simulink model "Simulator1"  (R2024a)
settings: Solver=VariableStepAuto  StartTime=0.0  StopTime=inf  RelTol=1e-5
values from neighbouring files (symbols this model uses):
  I = [3000 0 0 ... (first row only)    [Constants_gui.m]    (also in constants.m; mbi.m = [15, .25, .20; set_up_HW7.m = I-Id; setupConstantRateSDA.m)
  invI = inv(I)    [Constants_gui.m]    (also in constants.m; mbi.m; set_up_HW7.m; setupConstantRateSDA.m)
  q_init = q_init/norm(q_init)    [Constants_gui.m]    (also in constants.m = [-0.5 -0.5 -0.5 0.5]; mbi.m = [0 0 0 1]'; set_up_HW7.m = [0 0 0 1]'; setupConstantRateSDA.m)
  wbn_init = pi/30*[0 0 0]'    [Constants_gui.m]    (also in constants.m = pi/180 * [0.1; 0.2; 0.15]; mbi.m = [0 0 0]'; set_up_HW7.m = pi/30*[0 0 .01]'; setupConstantRateSDA.m)
  wn = 0.01    [Constants_gui.m]    (also in constants.m = 0.05; setupConstantRateSDA.m = 0.05)
  zet = .7071    (= 0.7071)    [Constants_gui.m]    (also in constants.m; setupConstantRateSDA.m)
undefined symbols (not defined in the file or in its folder): w_init
libraries: sharedtransform x5, aerolibutil x5, sharedutil x3, simulink x2, dspinverses x1
(part 4 of 4)

== system Simulator1/Mode 4: Slew1/ACS/Free Rigid Body /Quaternion Integration ==
  w_Body : Inport
  Integrator1 : Integrator  InitialCondition=q_init
  q_normalize : Subsystem
  qderiv : Subsystem
  q_I_Body : Outport
  wires:
  w_Body/1 -> qderiv/1(w)
  q_normalize/1(q_out) -> qderiv/2(q), q_I_Body/1
  Integrator1/1 -> q_normalize/1(q_in)
  qderiv/1(qd) -> Integrator1/1

== system Simulator1/Mode 4: Slew1/Subsystem/Quaternion Integration/q_normalize ==
  q_in : Inport  PortDimensions=4
  Dot Product : DotProduct  OutDataTypeStr=Inherit: Inherit via internal rule
  Product : Product  Inputs=*/  InputSameDT=on  SaturateOnIntegerOverflow=on  OutDataTypeStr=Inherit: Same as first input
  SignedSqrt : Sqrt  IntermediateResultsDataTypeStr=double
  q_out : Outport
  wires:
  Dot Product/1 -> SignedSqrt/1
  q_in/1 -> Product/1, Dot Product/1, Dot Product/2
  SignedSqrt/1 -> Product/2
  Product/1 -> q_out/1

== system Simulator1/Mode 4: Slew1/Subsystem/Quaternion Integration/qderiv ==
  w : Inport
  q : Inport  Port=2
  Mux : Mux  Inputs=2
  Mux1 : Mux
  qd1 : Fcn  Expr=(u(7)*u(1)-u(6)*u(2)+u(5)*u(3))/2
  qd2 : Fcn  Expr=(u(6)*u(1)+u(7)*u(2)-u(4)*u(3))/2
  qd3 : Fcn  Expr=(-u(5)*u(1)+u(4)*u(2)+u(7)*u(3))/2
  qd4 : Fcn  Expr=(-u(4)*u(1)-u(5)*u(2)-u(6)*u(3))/2
  qd : Outport
  wires:
  w/1 -> Mux/1
  q/1 -> Mux/2
  Mux/1 -> qd1/1, qd2/1, qd3/1, qd4/1
  qd1/1 -> Mux1/1
  qd2/1 -> Mux1/2
  qd3/1 -> Mux1/3
  qd4/1 -> Mux1/4
  Mux1/1 -> qd/1

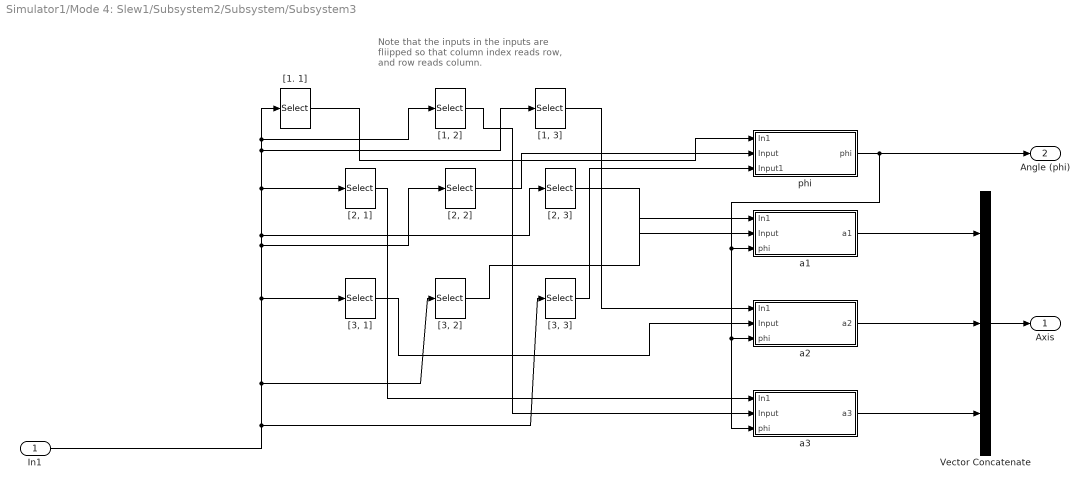
== system Simulator1/Mode 4: Slew1/Subsystem2/Subsystem/Subsystem3 ==
  note: Note that the inputs in the inputs are fliipped so that column index reads row, and row reads column.
  In1 : Inport
  Vector Concatenate : Concatenate  NumInputs=3
  "[1, 2]" : Selector  NumberOfDimensions=2  InputPortWidth=3  IndexOptions=Index vector (dialog),Index vector (dialog)  Indices=2,1  OutputSizes=1,1
  "[1, 3]" : Selector  NumberOfDimensions=2  InputPortWidth=3  IndexOptions=Index vector (dialog),Index vector (dialog)  Indices=3,1  OutputSizes=1,1
  "[1. 1]" : Selector  NumberOfDimensions=2  InputPortWidth=3  IndexOptions=Index vector (dialog),Index vector (dialog)  Indices=1,1  OutputSizes=1,1
  "[2, 1]" : Selector  NumberOfDimensions=2  InputPortWidth=3  IndexOptions=Index vector (dialog),Index vector (dialog)  Indices=1,2  OutputSizes=1,1
  "[2, 2]" : Selector  NumberOfDimensions=2  InputPortWidth=3  IndexOptions=Index vector (dialog),Index vector (dialog)  Indices=2,2  OutputSizes=1,1
  "[2, 3]" : Selector  NumberOfDimensions=2  InputPortWidth=3  IndexOptions=Index vector (dialog),Index vector (dialog)  Indices=3,2  OutputSizes=1,1
  "[3, 1]" : Selector  NumberOfDimensions=2  InputPortWidth=3  IndexOptions=Index vector (dialog),Index vector (dialog)  Indices=1,3  OutputSizes=1,1
  "[3, 2]" : Selector  NumberOfDimensions=2  InputPortWidth=3  IndexOptions=Index vector (dialog),Index vector (dialog)  Indices=2,3  OutputSizes=1,1
  "[3, 3]" : Selector  NumberOfDimensions=2  InputPortWidth=3  IndexOptions=Index vector (dialog),Index vector (dialog)  Indices=3,3  OutputSizes=1,1
  a1 : Subsystem
  a2 : Subsystem
  a3 : Subsystem
  phi : Subsystem
  Axis : Outport
  Angle (phi) : Outport  Port=2
  wires:
  a3/1(a3) -> Vector Concatenate/3
  Vector Concatenate/1 -> Axis/1
  a1/1(a1) -> Vector Concatenate/1
  "[2, 3]"/1 -> a1/2(Input)
  "[3, 3]"/1 -> phi/3(Input1)
  "[3, 1]"/1 -> a2/2(Input)
  "[1. 1]"/1 -> phi/1(In1)
  phi/1(phi) -> Angle (phi)/1, a3/3(phi), a2/3(phi), a1/3(phi)
  "[1, 2]"/1 -> a3/2(Input)
  a2/1(a2) -> Vector Concatenate/2
  "[2, 1]"/1 -> a3/1(In1)
  "[2, 2]"/1 -> phi/2(Input)
  "[3, 2]"/1 -> a1/1(In1)
  "[1, 3]"/1 -> a2/1(In1)
  In1/1 -> "[3, 2]"/1, "[3, 1]"/1, "[2, 1]"/1, "[1, 3]"/1, "[1, 2]"/1, "[1. 1]"/1, "[2, 3]"/1, "[2, 2]"/1, "[3, 3]"/1

== system Simulator1/Mode 4: Slew1/Subsystem2/Subsystem/w (q1,q2,q3,q0) to (q0,q1,q2,q3)  ==
  y : Inport
  Vector Concatenate : Concatenate
  e_q_vect1 : Selector  InputPortWidth=4  IndexOptions=Index vector (dialog)  Indices=[1 2 3]  OutputSizes=1
  e_q_vect2 : Selector  InputPortWidth=4  IndexOptions=Index vector (dialog)  Indices=[4]  OutputSizes=1
  Out1 : Outport
  wires:
  Vector Concatenate/1 -> Out1/1
  e_q_vect1/1 -> Vector Concatenate/2
  e_q_vect2/1 -> Vector Concatenate/1
  y/1 -> e_q_vect1/1, e_q_vect2/1

== system Simulator1/Mode 5: Attitude Control/Free Rigid Body /Quaternion Integration/q_normalize ==
  q_in : Inport  PortDimensions=4
  Dot Product : DotProduct  OutDataTypeStr=Inherit: Inherit via internal rule
  Product : Product  Inputs=*/  InputSameDT=on  SaturateOnIntegerOverflow=on  OutDataTypeStr=Inherit: Same as first input
  SignedSqrt : Sqrt  IntermediateResultsDataTypeStr=double
  q_out : Outport
  wires:
  Product/1 -> q_out/1
  SignedSqrt/1 -> Product/2
  q_in/1 -> Dot Product/2, Dot Product/1, Product/1
  Dot Product/1 -> SignedSqrt/1

== system Simulator1/Mode 5: Attitude Control/Free Rigid Body /Quaternion Integration/qderiv ==
  w : Inport
  q : Inport  Port=2
  Mux : Mux  Inputs=2
  Mux1 : Mux
  qd1 : Fcn  Expr=(u(7)*u(1)-u(6)*u(2)+u(5)*u(3))/2
  qd2 : Fcn  Expr=(u(6)*u(1)+u(7)*u(2)-u(4)*u(3))/2
  qd3 : Fcn  Expr=(-u(5)*u(1)+u(4)*u(2)+u(7)*u(3))/2
  qd4 : Fcn  Expr=(-u(4)*u(1)-u(5)*u(2)-u(6)*u(3))/2
  qd : Outport
  wires:
  Mux1/1 -> qd/1
  qd4/1 -> Mux1/4
  qd3/1 -> Mux1/3
  qd2/1 -> Mux1/2
  qd1/1 -> Mux1/1
  Mux/1 -> qd4/1, qd3/1, qd2/1, qd1/1
  q/1 -> Mux/2
  w/1 -> Mux/1

== system Simulator1/Mode 4: Slew1/ACS/Free Rigid Body /Quaternion Integration/q_normalize ==
  q_in : Inport  PortDimensions=4
  Dot Product : DotProduct  OutDataTypeStr=Inherit: Inherit via internal rule
  Product : Product  Inputs=*/  InputSameDT=on  SaturateOnIntegerOverflow=on  OutDataTypeStr=Inherit: Same as first input
  SignedSqrt : Sqrt  IntermediateResultsDataTypeStr=double
  q_out : Outport
  wires:
  Product/1 -> q_out/1
  SignedSqrt/1 -> Product/2
  q_in/1 -> Dot Product/2, Dot Product/1, Product/1
  Dot Product/1 -> SignedSqrt/1

== system Simulator1/Mode 4: Slew1/ACS/Free Rigid Body /Quaternion Integration/qderiv ==
  w : Inport
  q : Inport  Port=2
  Mux : Mux  Inputs=2
  Mux1 : Mux
  qd1 : Fcn  Expr=(u(7)*u(1)-u(6)*u(2)+u(5)*u(3))/2
  qd2 : Fcn  Expr=(u(6)*u(1)+u(7)*u(2)-u(4)*u(3))/2
  qd3 : Fcn  Expr=(-u(5)*u(1)+u(4)*u(2)+u(7)*u(3))/2
  qd4 : Fcn  Expr=(-u(4)*u(1)-u(5)*u(2)-u(6)*u(3))/2
  qd : Outport
  wires:
  Mux1/1 -> qd/1
  qd4/1 -> Mux1/4
  qd3/1 -> Mux1/3
  qd2/1 -> Mux1/2
  qd1/1 -> Mux1/1
  Mux/1 -> qd4/1, qd3/1, qd2/1, qd1/1
  q/1 -> Mux/2
  w/1 -> Mux/1

== system Simulator1/Mode 4: Slew1/Subsystem2/Subsystem/Subsystem3/a1 ==
  In1 : Inport
  Input : Inport  Port=2
  phi : Inport  Port=3
  Divide : Product  Inputs=*/
  Minus : Sum  Inputs=+-
  Multiply : Gain  Gain=2
  Sin : Trigonometry
  a1 : Outport
  wires:
  In1/1 -> Minus/1
  Input/1 -> Minus/2
  phi/1 -> Sin/1
  Sin/1 -> Multiply/1
  Minus/1 -> Divide/1
  Divide/1 -> a1/1
  Multiply/1 -> Divide/2

== system Simulator1/Mode 4: Slew1/Subsystem2/Subsystem/Subsystem3/a2 ==
  In1 : Inport
  Input : Inport  Port=2
  phi : Inport  Port=3
  Divide : Product  Inputs=*/
  Minus : Sum  Inputs=+-
  Multiply : Gain  Gain=2
  Sin : Trigonometry
  a2 : Outport
  wires:
  In1/1 -> Minus/1
  Input/1 -> Minus/2
  phi/1 -> Sin/1
  Sin/1 -> Multiply/1
  Minus/1 -> Divide/1
  Divide/1 -> a2/1
  Multiply/1 -> Divide/2

== system Simulator1/Mode 4: Slew1/Subsystem2/Subsystem/Subsystem3/a3 ==
  In1 : Inport
  Input : Inport  Port=2
  phi : Inport  Port=3
  Divide : Product  Inputs=*/
  Minus : Sum  Inputs=+-
  Multiply : Gain  Gain=2
  Sin : Trigonometry
  a3 : Outport
  wires:
  In1/1 -> Minus/1
  Input/1 -> Minus/2
  phi/1 -> Sin/1
  Sin/1 -> Multiply/1
  Minus/1 -> Divide/1
  Divide/1 -> a3/1
  Multiply/1 -> Divide/2

== system Simulator1/Mode 4: Slew1/Subsystem2/Subsystem/Subsystem3/phi ==
  In1 : Inport
  Input : Inport  Port=2
  Input1 : Inport  Port=3
  Acos : Trigonometry  Operator=acos
  Add : Sum  Inputs=++++
  Constant : Constant  Value=-1
  Multiply : Gain  Gain=0.5
  phi : Outport
  wires:
  Input1/1 -> Add/3
  Input/1 -> Add/2
  In1/1 -> Add/1
  Constant/1 -> Add/4
  Add/1 -> Multiply/1
  Multiply/1 -> Acos/1
  Acos/1 -> phi/1
